simulink model "Commande_5_ReglageCascade_Action_Integrale"  (R2015a)
settings: Solver=ode45  StartTime=0.0  StopTime=20  FixedStep=0.001  RelTol=1e-3
values from neighbouring files (symbols this model uses):
  Kd = p1^2*J4    (= 0.0333)    [A_1_Data.m]    (also in matlab.mat = 0.009)
  Kp = -2*p1*J4    (= 0.00222)    [A_1_Data.m]    (also in matlab.mat = 0.0006)
  s = tf('s')    [A_3_LoopShaping.m]    (also in A_4_Hinfini.m = zpk('s'))
  X = [0;0;0;0;0;0;0;0]    [A_1_Data.m]
  Y = [0;0;0;0;0;0;0;0]    [A_1_Data.m]
undefined symbols (not defined in the file or in its folder): sfun3d, Z
libraries: sm_lib x331, nesl_utility x15, simulink x1
(part 10 of 10)

== matlab function Commande_5_ReglageCascade_Action_Integrale/Regulateur de la partie mecanique/MATLAB Function ==
  data: Q input; R input; E input; DX1 input; DX2 input; V output
function V= fcn(Q,R,E,DX1,DX2)

Qd1 = Q(1,1) ;Rd1=R(1,1) ;
Qd2 = Q(2,2) ;Rd2=R(2,2) ;
Qd3 = Q(3,3) ;Rd3=R(3,3) ;

% Les poles du systeme entier:
%s1 = -7 ; s2 =-15 ;
s1 = -20 ; s2 =-30 ; s3 =2*(s1+s2) ;
b = -(s1+s2+s3); c = s1*s2+s1*s3+s2*s3;
% les poles du retour d'etat:
p1=(-b + sqrt(b^2-4*c))/2 ;p2=(-b - sqrt(b^2-4*c))/2;
Ks=-s1*s2*s3 ;
% Regulateur 1
K11 = Qd1 + p1*p2;
K21 = Rd1 - (p1+p2) ;
 v1=-K11*DX1(1) - K21*DX2(1) + Ks*E(1);
%Regulateur 2
K12 = Qd2 + p1*p2;
K22 = Rd2 - (p1+p2) ;
 v2=-K12*DX1(2) - K22*DX2(2) + Ks*E(2);
%Regulateur 3
K13 = Qd3 + p1*p2;
K23 = Rd3 - (p1+p2) ;
v3=-K13*DX1(3) - K23*DX2(3) + Ks*E(3);
% Clacule de V ;
V= [v1;v2;v3] ;

== matlab function Commande_5_ReglageCascade_Action_Integrale/Regulateur de la partie electrique/Calcule de gains1 ==
  data: e input; ei output; ep output
function [ei , ep]= fcn(e)

b1 = -1.1250e+03 ;
Ki=0.119;
% ei  :c'est l'erreur du couple multiplie par le gain de l'integrateur KI(du
% regulateur)
% ei  :c'est l'erreur du couple multiplie par le gain proportinnel Kp (du
% regulateur)

% le pole desire :
p = 1.5*b1;
Kp= -p/Ki ;
KI = -b1*Kp ;
ep = e*Kp ;
ei = e*KI ;

% Remarque ;
% Ki:constante du couple (couple=Ki*courant)
% KI : pour l'action integrale

== matlab function Commande_5_ReglageCascade_Action_Integrale/Regulateur de la partie electrique/Decoupleur Tension Vitess ==
  data: DUd input; DU output; DX2 input
function DU = fcn(DUd,DX2)


b2 = -99.4718 ;
b3 =833.3333 ;

DU = (DUd - b2*DX2)/b3 ;
